simulink model "ekf2"  (R2023b)
settings: Solver=VariableStepAuto  StartTime=0.0  StopTime=Tend_slk  RelTol=1e-3
values from neighbouring files (symbols this model uses):
  IMU_w_b_bias = IMU_var_bias_matrix(:,2)    [ekf1_script.m]    (also in ekf2_script.m; ekf3_script.m)
  meas_pole = 15    [ekf1_script.m]    (also in ekf2_script.m; ekf3_script.m)
  P0_phth = diag([P0_ph,P0_th,P0_bias_wp,P0_bias_wq,P0_bias_wr])    [ekf2_script.m]    (also in ekf3_script.m)
  P0_ps = 100    [complementary_filter_script.m]    (also in ekf1_script.m; ekf2_script.m; ekf3_script.m)
  Q_phth = diag([q_ph,q_th,q_bias_w_b,q_bias_w_b,q_bias_w_b])    [ekf2_script.m]    (also in ekf3_script.m)
  q_ps = 100e-0    (= 100)    [complementary_filter_script.m]    (also in ekf1_script.m = 200; ekf2_script.m = 170; ekf3_script.m = 170)
  R_phth = diag([r_ph,r_th])    [ekf2_script.m]    (also in ekf3_script.m)
  r_ps = 600e+0    (= 600)    [complementary_filter_script.m]    (also in ekf1_script.m = 170; ekf2_script.m = 200; ekf3_script.m = 200)
  Ts_EKF_integr = 0.001    [complementary_filter_script.m]    (also in ekf1_script.m = 0.0001; ekf2_script.m = 0.0001; ekf3_script.m = 0.0001)
  Ts_EKF_meas = 0.01    [complementary_filter_script.m]    (also in ekf1_script.m; ekf2_script.m; ekf3_script.m)
  Ts_slk = 0.01    [complementary_filter_script.m]    (also in ekf1_script.m; ekf2_script.m; ekf3_script.m)
  x0_phth = [ph0;th0;bias_wp0;bias_wq0;bias_wr0]    [ekf2_script.m]    (also in ekf3_script.m)
  x0_ps = 0    [complementary_filter_script.m]    (also in ekf2_script.m; ekf3_script.m)
settings Model: Creator=teoma  LastModifiedBy=teoma

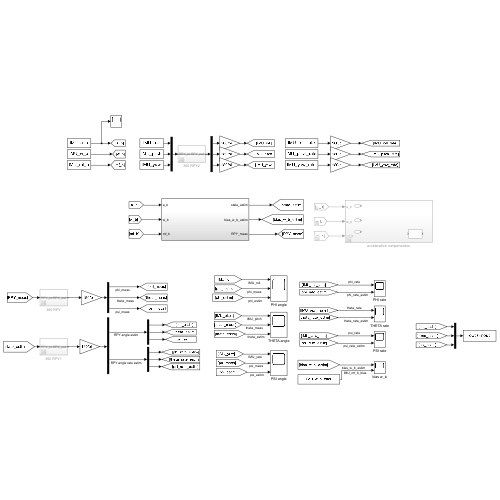
[thumbnail: Simulink's stored preview of the top-level diagram]
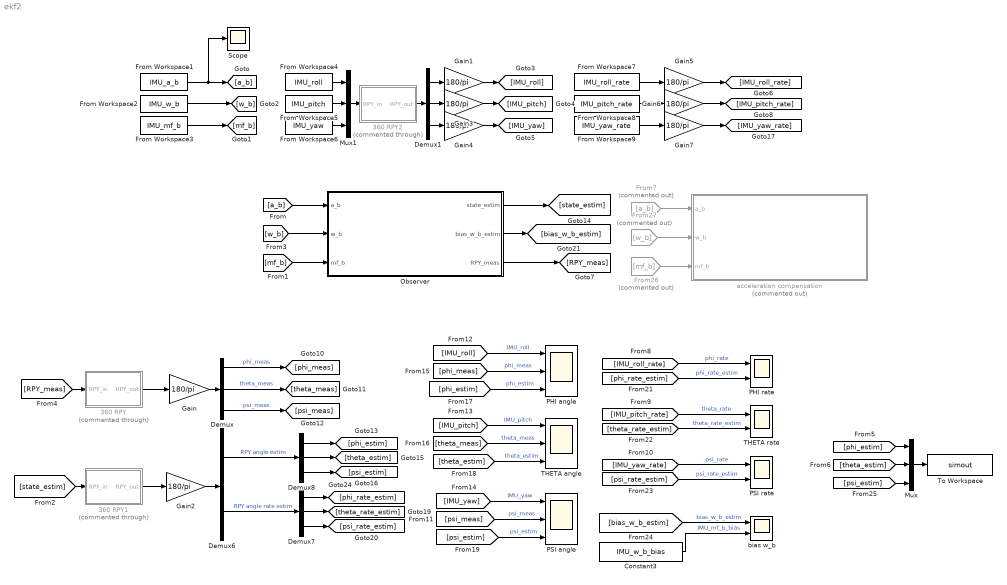
== system ekf2 ==
  360 RPY : Subsystem  Commented=through
  360 RPY1 : Subsystem  Commented=through
  360 RPY2 : Subsystem  Commented=through
  Constant3 : Constant  Value=IMU_w_b_bias
  Demux{,1,7..8} (4 alike) : Demux  Outputs=3
  Demux6 : Demux  Outputs=2
  From Workspace1 : FromWorkspace  VariableName=IMU_a_b  OutDataTypeStr=double  SampleTime=Ts_slk  Interpolate=off  OutputAfterFinalValue=Setting to zero
  From Workspace2 : FromWorkspace  VariableName=IMU_w_b  OutDataTypeStr=double  SampleTime=Ts_slk  Interpolate=off  OutputAfterFinalValue=Setting to zero
  From Workspace3 : FromWorkspace  VariableName=IMU_mf_b  OutDataTypeStr=double  SampleTime=Ts_slk  Interpolate=off  OutputAfterFinalValue=Setting to zero
  From Workspace4 : FromWorkspace  VariableName=IMU_roll  OutDataTypeStr=double  SampleTime=Ts_slk  Interpolate=off  OutputAfterFinalValue=Setting to zero
  From Workspace5 : FromWorkspace  VariableName=IMU_pitch  OutDataTypeStr=double  SampleTime=Ts_slk  Interpolate=off  OutputAfterFinalValue=Setting to zero
  From Workspace6 : FromWorkspace  VariableName=IMU_yaw  OutDataTypeStr=double  SampleTime=Ts_slk  Interpolate=off  OutputAfterFinalValue=Setting to zero
  From Workspace7 : FromWorkspace  VariableName=IMU_roll_rate  OutDataTypeStr=double  SampleTime=Ts_slk  Interpolate=off  OutputAfterFinalValue=Setting to zero
  From Workspace8 : FromWorkspace  VariableName=IMU_pitch_rate  OutDataTypeStr=double  SampleTime=Ts_slk  Interpolate=off  OutputAfterFinalValue=Setting to zero
  From Workspace9 : FromWorkspace  VariableName=IMU_yaw_rate  OutDataTypeStr=double  SampleTime=Ts_slk  Interpolate=off  OutputAfterFinalValue=Setting to zero
  From26 : From  Commented=on  GotoTag=mf_b
  From27 : From  Commented=on  GotoTag=w_b
  From7 : From  Commented=on  GotoTag=a_b
  Gain{,1..7} (8 alike) : Gain  Gain=180/pi
  Mux : Mux  Inputs=3
  Mux1 : Mux  Inputs=3
  Observer : Subsystem
  PHI angle : Scope  NumInputPorts=3
  PHI rate : Scope  NumInputPorts=2
  PSI angle : Scope  NumInputPorts=3
  PSI rate : Scope  NumInputPorts=2
  Scope : Scope
  THETA angle : Scope  NumInputPorts=3
  THETA rate : Scope  NumInputPorts=2
  To Workspace : ToWorkspace  VariableName=simout  SampleTime=-1
  acceleration compensation : Subsystem  Commented=on
  bias w_b : Scope  NumInputPorts=2
  wires:
  [a_b] -> Observer/1(a_b)
  Gain6/1 -> [IMU_pitch_rate]
  Observer/2(bias_w_b_estim) -> [bias_w_b_estim]
  [mf_b] -> Observer/3(mf_b)
  [IMU_roll] -> PHI angle/1  "IMU_roll"
  From Workspace9/1 -> Gain7/1
  Observer/3(RPY_meas) -> [RPY_meas]
  [IMU_yaw_rate] -> PSI rate/1  "psi_rate"
  [psi_estim] -> PSI angle/3  "psi_estim"
  Observer/1(state_estim) -> [state_estim]
  [w_b] -> Observer/2(w_b)
  From Workspace2/1 -> [w_b]
  [theta_estim] -> THETA angle/3  "theta_estim"
  [IMU_roll_rate] -> PHI rate/1  "phi_rate"
  [phi_meas] -> PHI angle/2  "phi_meas"
  Constant3/1 -> bias w_b/2  "IMU_mf_b_bias"
  From Workspace1/1 -> [a_b], Scope/1
  From Workspace7/1 -> Gain5/1
  [IMU_yaw] -> PSI angle/1  "IMU_yaw"
  [phi_estim] -> PHI angle/3  "phi_estim"
  [theta_rate_estim] -> THETA rate/2  "theta_rate_estim"
  [psi_rate_estim] -> PSI rate/2  "psi_rate_estim"
  [IMU_pitch_rate] -> THETA rate/1  "theta_rate"
  Gain7/1 -> [IMU_yaw_rate]
  [theta_meas] -> THETA angle/2  "theta_meas"
  [IMU_pitch] -> THETA angle/1  "IMU_pitch"
  [psi_meas] -> PSI angle/2  "psi_meas"
  Gain5/1 -> [IMU_roll_rate]
  From Workspace8/1 -> Gain6/1
  [phi_rate_estim] -> PHI rate/2  "phi_rate_estim"
  From Workspace3/1 -> [mf_b]
  [bias_w_b_estim] -> bias w_b/1  "bias_w_b_estim"
  Mux/1 -> To Workspace/1
  [phi_estim] -> Mux/1
  [theta_estim] -> Mux/2
  [psi_estim] -> Mux/3
  From27/1 -> acceleration compensation/2(w_b)
  From26/1 -> acceleration compensation/3(mf_b)
  From7/1 -> acceleration compensation/1(a_b)
  360 RPY1/1(RPY_out) -> Gain2/1
  Demux6/1 -> Demux8/1  "RPY angle estim"
  Demux6/2 -> Demux7/1  "RPY angle rate estim"
  Demux/2 -> [theta_meas]  "theta_meas"
  Gain/1 -> Demux/1
  Demux7/2 -> [theta_rate_estim]
  Demux8/3 -> [psi_estim]
  Demux8/2 -> [theta_estim]
  Demux7/3 -> [psi_rate_estim]
  Demux/1 -> [phi_meas]  "phi_meas"
  Gain2/1 -> Demux6/1
  Demux8/1 -> [phi_estim]
  Demux7/1 -> [phi_rate_estim]
  360 RPY/1(RPY_out) -> Gain/1
  Demux/3 -> [psi_meas]  "psi_meas"
  [state_estim] -> 360 RPY1/1(RPY_in)
  [RPY_meas] -> 360 RPY/1(RPY_in)
  Mux1/1 -> 360 RPY2/1(RPY_in)
  Demux1/1 -> Gain1/1
  From Workspace4/1 -> Mux1/1
  Gain1/1 -> [IMU_roll]
  Gain3/1 -> [IMU_pitch]
  Demux1/2 -> Gain3/1
  Demux1/3 -> Gain4/1
  From Workspace5/1 -> Mux1/2
  Gain4/1 -> [IMU_yaw]
  From Workspace6/1 -> Mux1/3
  360 RPY2/1(RPY_out) -> Demux1/1

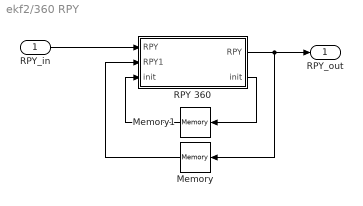
== system ekf2/360 RPY ==
  RPY_in : Inport
  Memory : Memory
  Memory1 : Memory
  RPY 360 : MATLAB Function  TreatAsAtomicUnit=on
  RPY_out : Outport
  wires:
  Memory/1 -> RPY 360/2(RPY1)
  Memory1/1 -> RPY 360/3("init ")
  RPY 360/2(init) -> Memory1/1
  RPY 360/1(RPY) -> Memory/1, RPY_out/1
  RPY_in/1 -> RPY 360/1("RPY ")

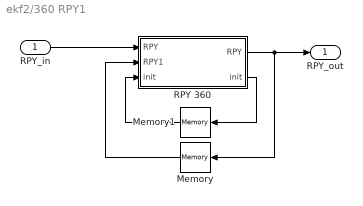
== system ekf2/360 RPY1 ==
  RPY_in : Inport
  Memory : Memory
  Memory1 : Memory
  RPY 360 : MATLAB Function  TreatAsAtomicUnit=on
  RPY_out : Outport
  wires:
  Memory/1 -> RPY 360/2(RPY1)
  Memory1/1 -> RPY 360/3("init ")
  RPY 360/2(init) -> Memory1/1
  RPY 360/1(RPY) -> Memory/1, RPY_out/1
  RPY_in/1 -> RPY 360/1("RPY ")

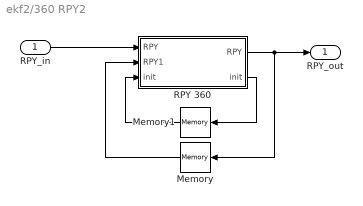
== system ekf2/360 RPY2 ==
  RPY_in : Inport
  Memory : Memory
  Memory1 : Memory
  RPY 360 : MATLAB Function  TreatAsAtomicUnit=on
  RPY_out : Outport
  wires:
  Memory/1 -> RPY 360/2(RPY1)
  Memory1/1 -> RPY 360/3("init ")
  RPY 360/2(init) -> Memory1/1
  RPY 360/1(RPY) -> Memory/1, RPY_out/1
  RPY_in/1 -> RPY 360/1("RPY ")

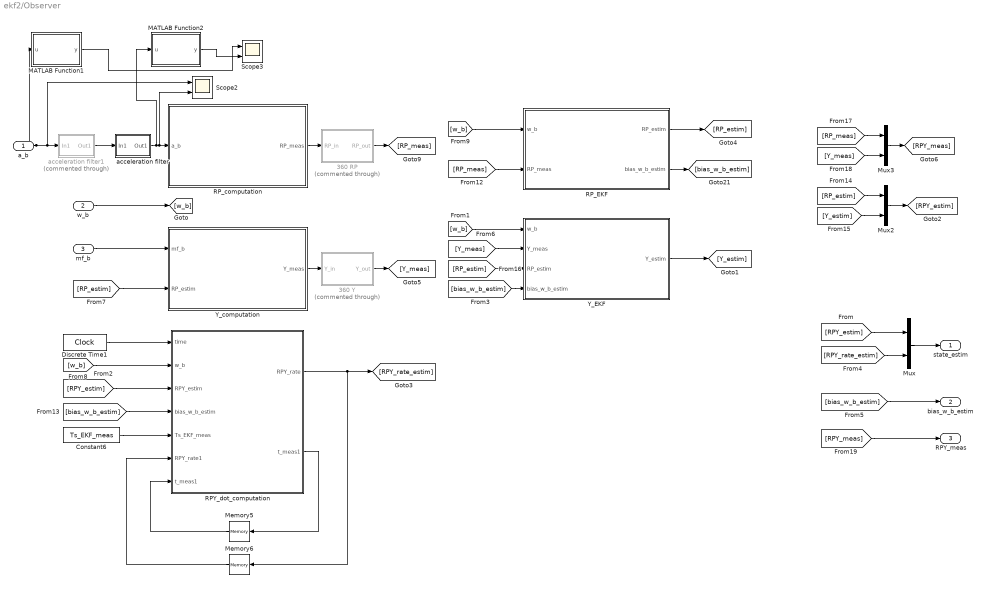
== system ekf2/Observer ==
  a_b : Inport
  w_b : Inport  Port=2
  mf_b : Inport  Port=3
  360 RP : Subsystem  Commented=through
  360 Y : Subsystem  Commented=through
  Constant6 : Constant  Value=Ts_EKF_meas
  Discrete Time1 : DigitalClock  SampleTime=Ts_slk
  MATLAB Function1 : MATLAB Function  TreatAsAtomicUnit=on
  MATLAB Function2 : MATLAB Function  TreatAsAtomicUnit=on
  Memory5 : Memory
  Memory6 : Memory
  Mux : Mux  Inputs=2
  Mux2 : Mux  Inputs=2
  Mux3 : Mux  Inputs=2
  RPY_dot_computation : MATLAB Function  TreatAsAtomicUnit=on
  RP_EKF : Subsystem
  RP_computation : MATLAB Function  TreatAsAtomicUnit=on
  Scope2 : Scope  NumInputPorts=2
  Scope3 : Scope  NumInputPorts=2
  Y_EKF : Subsystem
  Y_computation : MATLAB Function  TreatAsAtomicUnit=on
  acceleration filter : Subsystem  mask{p=meas_pole}
      mask prompts: p "pole (p)"
  acceleration filter1 : Subsystem  Commented=through  mask{p=5}
      mask prompts: p "pole (p)"
  state_estim : Outport
  bias_w_b_estim : Outport  Port=2
  RPY_meas : Outport  Port=3
  wires:
  Memory5/1 -> RPY_dot_computation/7("t_meas1 ")
  Discrete Time1/1 -> RPY_dot_computation/1(time)
  RPY_dot_computation/2(t_meas1) -> Memory5/1
  [w_b] -> RPY_dot_computation/2(w_b)
  Memory6/1 -> RPY_dot_computation/6(RPY_rate1)
  RPY_dot_computation/1(RPY_rate) -> Memory6/1, [RPY_rate_estim]
  Constant6/1 -> RPY_dot_computation/5(Ts_EKF_meas)
  [RPY_estim] -> RPY_dot_computation/3(RPY_estim)
  [bias_w_b_estim] -> RPY_dot_computation/4(bias_w_b_estim)
  [RPY_estim] -> Mux/1
  [RPY_rate_estim] -> Mux/2
  Mux/1 -> state_estim/1
  [bias_w_b_estim] -> bias_w_b_estim/1
  [RPY_meas] -> RPY_meas/1
  RP_EKF/2(bias_w_b_estim) -> [bias_w_b_estim]
  [RP_estim] -> Y_computation/2(RP_estim)
  [Y_meas] -> Y_EKF/2(Y_meas)
  Y_computation/1(Y_meas) -> 360 Y/1(Y_in)
  RP_EKF/1(RP_estim) -> [RP_estim]
  [w_b] -> Y_EKF/1(w_b)
  RP_computation/1(RP_meas) -> 360 RP/1(RP_in)
  [RP_meas] -> RP_EKF/2(RP_meas)
  [w_b] -> RP_EKF/1(w_b)
  Y_EKF/1(Y_estim) -> [Y_estim]
  mf_b/1 -> Y_computation/1(mf_b)
  w_b/1 -> [w_b]
  [bias_w_b_estim] -> Y_EKF/4(bias_w_b_estim)
  [RP_estim] -> Mux2/1
  [Y_estim] -> Mux2/2
  Mux2/1 -> [RPY_estim]
  [RP_estim] -> Y_EKF/3(RP_estim)
  [RP_meas] -> Mux3/1
  Mux3/1 -> [RPY_meas]
  [Y_meas] -> Mux3/2
  MATLAB Function1/1(y) -> Scope3/1
  a_b/1 -> Scope2/1, acceleration filter1/1(In1), MATLAB Function1/1(u)
  MATLAB Function2/1(y) -> Scope3/2
  acceleration filter/1(Out1) -> MATLAB Function2/1(u), Scope2/2, RP_computation/1(a_b)
  360 Y/1(Y_out) -> [Y_meas]
  360 RP/1(RP_out) -> [RP_meas]
  acceleration filter1/1(Out1) -> acceleration filter/1(In1)

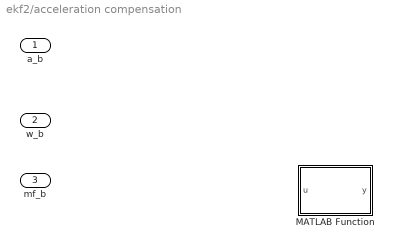
== system ekf2/acceleration compensation ==
  a_b : Inport
  w_b : Inport  Port=2
  mf_b : Inport  Port=3
  MATLAB Function : MATLAB Function  TreatAsAtomicUnit=on

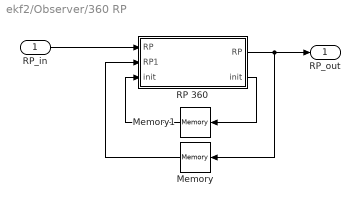
== system ekf2/Observer/360 RP ==
  RP_in : Inport
  Memory : Memory
  Memory1 : Memory
  RP 360 : MATLAB Function  TreatAsAtomicUnit=on
  RP_out : Outport
  wires:
  RP_in/1 -> RP 360/1("RP ")
  RP 360/1(RP) -> Memory/1, RP_out/1
  Memory/1 -> RP 360/2(RP1)
  RP 360/2(init) -> Memory1/1
  Memory1/1 -> RP 360/3("init ")

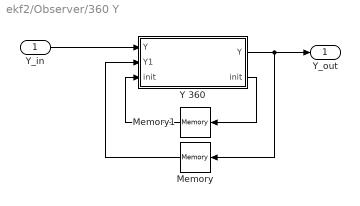
== system ekf2/Observer/360 Y ==
  Y_in : Inport
  Memory : Memory
  Memory1 : Memory
  Y 360 : MATLAB Function  TreatAsAtomicUnit=on
  Y_out : Outport
  wires:
  Y_in/1 -> Y 360/1("Y ")
  Y 360/1(Y) -> Memory/1, Y_out/1
  Memory/1 -> Y 360/2(Y1)
  Y 360/2(init) -> Memory1/1
  Memory1/1 -> Y 360/3("init ")

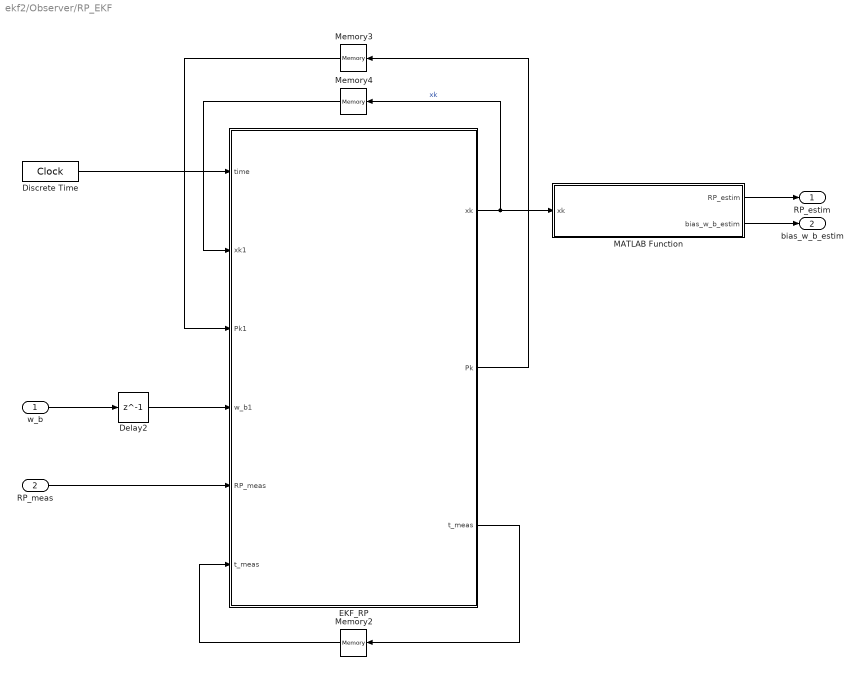
== system ekf2/Observer/RP_EKF ==
  w_b : Inport
  RP_meas : Inport  Port=2
  Delay2 : Delay  DelayLength=1  SampleTime=Ts_EKF_meas
  Discrete Time : DigitalClock  SampleTime=Ts_slk
  EKF_RP : MATLAB Function  TreatAsAtomicUnit=on
  MATLAB Function : MATLAB Function  TreatAsAtomicUnit=on
  Memory2 : Memory
  Memory3 : Memory  InitialCondition=P0_phth
  Memory4 : Memory  InitialCondition=x0_phth
  RP_estim : Outport
  bias_w_b_estim : Outport  Port=2
  wires:
  w_b/1 -> Delay2/1
  EKF_RP/2(Pk) -> Memory3/1
  Memory2/1 -> EKF_RP/6("t_meas ")
  EKF_RP/3(t_meas) -> Memory2/1
  RP_meas/1 -> EKF_RP/5(RP_meas)
  Discrete Time/1 -> EKF_RP/1(time)
  Memory3/1 -> EKF_RP/3(Pk1)
  Delay2/1 -> EKF_RP/4(w_b1)
  Memory4/1 -> EKF_RP/2(xk1)
  EKF_RP/1(xk) -> Memory4/1, MATLAB Function/1(xk)  "xk"
  MATLAB Function/1(RP_estim) -> RP_estim/1
  MATLAB Function/2(bias_w_b_estim) -> bias_w_b_estim/1

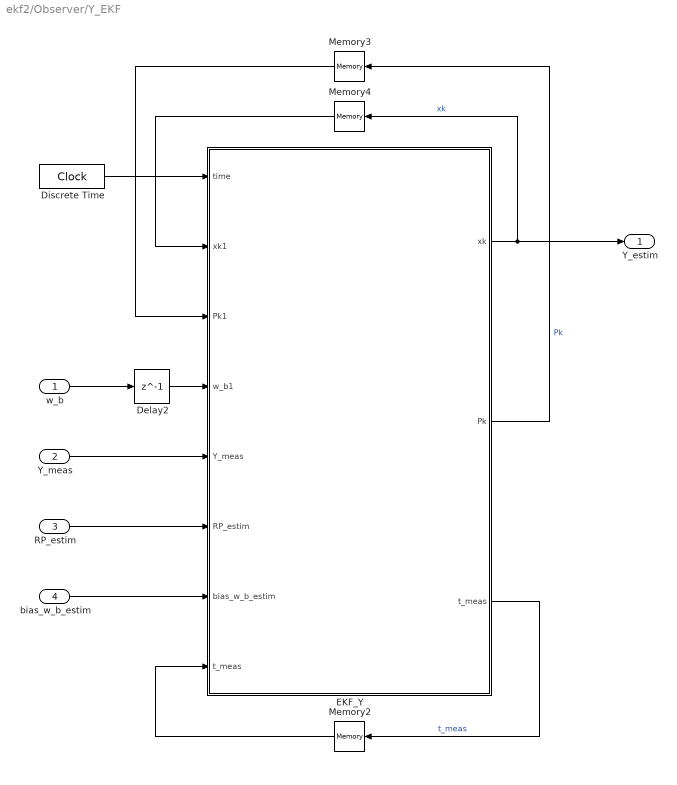
== system ekf2/Observer/Y_EKF ==
  w_b : Inport
  Y_meas : Inport  Port=2
  RP_estim : Inport  Port=3
  bias_w_b_estim : Inport  Port=4
  Delay2 : Delay  DelayLength=1  SampleTime=Ts_EKF_meas
  Discrete Time : DigitalClock  SampleTime=Ts_slk
  EKF_Y : MATLAB Function  TreatAsAtomicUnit=on
  Memory2 : Memory
  Memory3 : Memory  InitialCondition=ones(1,1)*P0_ps
  Memory4 : Memory  InitialCondition=ones(1,1)*x0_ps
  Y_estim : Outport
  wires:
  w_b/1 -> Delay2/1
  EKF_Y/2(Pk) -> Memory3/1  "Pk"
  Memory2/1 -> EKF_Y/8("t_meas ")
  EKF_Y/3(t_meas) -> Memory2/1  "t_meas"
  Y_meas/1 -> EKF_Y/5(Y_meas)
  Discrete Time/1 -> EKF_Y/1(time)
  Memory3/1 -> EKF_Y/3(Pk1)
  Delay2/1 -> EKF_Y/4(w_b1)
  Memory4/1 -> EKF_Y/2(xk1)
  EKF_Y/1(xk) -> Memory4/1, Y_estim/1  "xk"
  bias_w_b_estim/1 -> EKF_Y/7(bias_w_b_estim)
  RP_estim/1 -> EKF_Y/6(RP_estim)

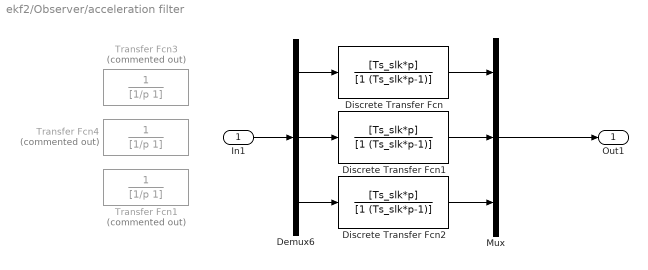
== system ekf2/Observer/acceleration filter ==
  In1 : Inport
  Demux6 : Demux  Outputs=3
  Discrete Transfer Fcn : DiscreteTransferFcn  Numerator=[Ts_slk*p]  Denominator=[1 (Ts_slk*p-1)]
  Discrete Transfer Fcn1 : DiscreteTransferFcn  Numerator=[Ts_slk*p]  Denominator=[1 (Ts_slk*p-1)]
  Discrete Transfer Fcn2 : DiscreteTransferFcn  Numerator=[Ts_slk*p]  Denominator=[1 (Ts_slk*p-1)]
  Mux : Mux  Inputs=3
  Transfer Fcn1 : TransferFcn  Commented=on  Denominator=[1/p 1]
  Transfer Fcn3 : TransferFcn  Commented=on  Denominator=[1/p 1]
  Transfer Fcn4 : TransferFcn  Commented=on  Denominator=[1/p 1]
  Out1 : Outport
  wires:
  Discrete Transfer Fcn1/1 -> Mux/2
  Demux6/3 -> Discrete Transfer Fcn2/1
  Mux/1 -> Out1/1
  Discrete Transfer Fcn2/1 -> Mux/3
  Discrete Transfer Fcn/1 -> Mux/1
  In1/1 -> Demux6/1
  Demux6/1 -> Discrete Transfer Fcn/1
  Demux6/2 -> Discrete Transfer Fcn1/1

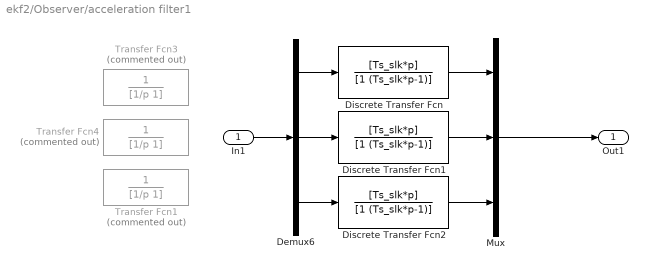
== system ekf2/Observer/acceleration filter1 ==
  In1 : Inport
  Demux6 : Demux  Outputs=3
  Discrete Transfer Fcn : DiscreteTransferFcn  Numerator=[Ts_slk*p]  Denominator=[1 (Ts_slk*p-1)]
  Discrete Transfer Fcn1 : DiscreteTransferFcn  Numerator=[Ts_slk*p]  Denominator=[1 (Ts_slk*p-1)]
  Discrete Transfer Fcn2 : DiscreteTransferFcn  Numerator=[Ts_slk*p]  Denominator=[1 (Ts_slk*p-1)]
  Mux : Mux  Inputs=3
  Transfer Fcn1 : TransferFcn  Commented=on  Denominator=[1/p 1]
  Transfer Fcn3 : TransferFcn  Commented=on  Denominator=[1/p 1]
  Transfer Fcn4 : TransferFcn  Commented=on  Denominator=[1/p 1]
  Out1 : Outport
  wires:
  Discrete Transfer Fcn1/1 -> Mux/2
  Demux6/3 -> Discrete Transfer Fcn2/1
  Mux/1 -> Out1/1
  Discrete Transfer Fcn2/1 -> Mux/3
  Discrete Transfer Fcn/1 -> Mux/1
  In1/1 -> Demux6/1
  Demux6/1 -> Discrete Transfer Fcn/1
  Demux6/2 -> Discrete Transfer Fcn1/1

== matlab function ekf2/Observer/RP_EKF/MATLAB Function ==
  data: xk input; RP_estim output; bias_w_b_estim output
function [RP_estim, bias_w_b_estim] = state_extraction(xk)

RP_estim        = xk(1:2,1);
bias_w_b_estim  = xk(3:5,1);
end

== matlab function ekf2/acceleration compensation/MATLAB Function ==
  data: u input; y output
function y = GCF(u)

y = u;

== matlab function ekf2/360 RPY2/RPY 360 ==
  data: RPY input; RPY output; RPY1 input; init output; init input
function [RPY,init] = RPY_360(RPY,RPY1,init)
if init < 2 
    if init == 0
        init = 1;
        RPY1 = RPY;
    elseif init == 1
        if (RPY - RPY1)'*(RPY - RPY1) > 0.01
            init = 2;
            RPY1 = RPY;
        end
    end
end

% - pi <= PHI <= + pi PHI uses atan2()
if abs(RPY(1) - RPY1(1)) > pi*0.99
    RPY(1) = RPY(1) + sign(RPY1(1))*(2*pi);
end
% - pi/2 <= THETA <= + pi/2 THETA uses asin()
if abs(RPY(2) - RPY1(2)) > pi/2*0.99
    RPY(2) = RPY(2) + sign(RPY1(2))*(2*pi);
end
% - pi <= PSI <= + pi PSI uses atan2()
if abs(RPY(3) - RPY1(3)) > pi*0.99
    RPY(3) = RPY(3) + sign(RPY1(3))*(2*pi);
end
end

== matlab function ekf2/Observer/RPY_dot_computation ==
  data: time input; w_b input; RPY_estim input; bias_w_b_estim input; Ts_EKF_meas input; RPY_rate1 input; RPY_rate output; t_meas1 input; t_meas1 output
function [RPY_rate,t_meas1] = RPY_dot_computation(time,w_b,RPY_estim,bias_w_b_estim,Ts_EKF_meas,RPY_rate1,t_meas1)

if time - t_meas1 >= Ts_EKF_meas || time == 0
    wp          =       w_b(1,1);               % p-dir of angular velocity w
    wq          =       w_b(2,1);               % q-dir of angular velocity w
    wr          =       w_b(3,1);               % r-dir of angular velocity w

    phi         =       RPY_estim(1,1);         % roll angle (rad)
    theta       =       RPY_estim(2,1);         % pitch angle (rad)
    psi         =       RPY_estim(3,1);         % yaw angle (rad)  
    bias_wp     =       bias_w_b_estim(1,1)*0;    % bias of p-dir of angular velocity w
    bias_wq     =       bias_w_b_estim(2,1)*0;    % bias of q-dir of angular velocity w
    bias_wr     =       bias_w_b_estim(3,1)*0;   % bias of r-dir of angular velocity w

    cph         =       cos(phi);
    cth         =       cos(theta);
    cps         =       cos(psi);
    sph         =       sin(phi);
    sth         =       sin(theta);
    sps         =       sin(psi);
    tth         =       sth/cth;

    % integration step
    t_meas1 = time;
    W_eta = [1,    sph*tth,    cph*tth;
             0,    cph,        -sph;
             0,    sph/cth,    cph/cth;];
    w_b_corrected = [wp-bias_wp; wq-bias_wq; wr-bias_wr;];
    RPY_rate = W_eta*w_b_corrected;
else
    RPY_rate = RPY_rate1;
end
end

== matlab function ekf2/360 RPY/RPY 360 ==
  data: RPY input; RPY output; RPY1 input; init output; init input
function [RPY,init] = RPY_360(RPY,RPY1,init)
if init < 2 
    if init == 0
        init = 1;
        RPY1 = RPY;
    elseif init == 1
        if (RPY - RPY1)'*(RPY - RPY1) > 0.01
            init = 2;
            RPY1 = RPY;
        end
    end
end

% - pi <= PHI <= + pi PHI uses atan2()
if abs(RPY(1) - RPY1(1)) > pi*0.99
    RPY(1) = RPY(1) + sign(RPY1(1))*(2*pi);
end
% - pi/2 <= THETA <= + pi/2 THETA uses asin()
if abs(RPY(2) - RPY1(2)) > pi/2*0.99
    RPY(2) = RPY(2) + sign(RPY1(2))*(2*pi);
end
% - pi <= PSI <= + pi PSI uses atan2()
if abs(RPY(3) - RPY1(3)) > pi*0.99
    RPY(3) = RPY(3) + sign(RPY1(3))*(2*pi);
end
end

== matlab function ekf2/Observer/360 Y/Y 360 ==
  data: Y input; Y output; Y1 input; init output; init input
function [Y,init] = Y_360(Y,Y1, init)
if init < 2 
    if init == 0
        init = 1;
        Y1 = Y;
    elseif init == 1
        if (Y - Y1)'*(Y - Y1) > 0.01
            init = 2;
            Y1 = Y;
        end
    end
end

% - pi <= PSI <= + pi PSI uses atan2()
if abs(Y - Y1) > pi*0.99
    Y = Y + sign(Y1)*(2*pi);
end

== matlab function ekf2/Observer/360 RP/RP 360 ==
  data: RP input; RP output; RP1 input; init output; init input
function [RP,init] = RP_360(RP,RP1, init)
if init < 2 
    if init == 0
        init = 1;
        RP1 = RP;
    elseif init == 1
        if (RP - RP1)'*(RP - RP1) > 0.01
            init = 2;
            RP1 = RP;
        end
    end
end

% - pi <= PHI <= + pi PHI uses atan2()
if abs(RP(1) - RP1(1)) > pi*0.99
    RP(1) = RP(1) + sign(RP1(1))*(2*pi);
end
% - pi/2 <= THETA <= + pi/2 THETA uses asin()
if abs(RP(2) - RP1(2)) > pi/2*0.99
    RP(2) = RP(2) + sign(RP1(2))*(2*pi);
end

end

== matlab function ekf2/Observer/Y_computation ==
  data: mf_b input; RP_estim input; Y_meas output
function Y_meas    = Y_computation(mf_b,RP_estim)
% description:
% - a_b             = measured linear acceleration in body-frame
% - w_b             = measured angular velocity in body-frame
% - mf_b            = measured magnetic field in body-frame
% - mf              = measured magnetic field in body-inertia
% - a_b_disturbe    = linear velocity measurement-noise
% - w_b_disturbe    = angular velocity measurement-noise
% - mf_b_disturbe   = magnetic field measurement-noise

% -------------------------------------------------------------------------------------------
% observation: the following computation works only if the angles
% phi,theta,psy are withing angles (-pi/2,+pi/2) (this is an open set, pi/2 is excluded)
% -------------------------------------------------------------------------------------------

ph_estim = RP_estim(1,1);
th_estim = RP_estim(2,1);

sph = sin(ph_estim);
cph = cos(ph_estim);

sth = sin(th_estim);
cth = cos(th_estim);

ps_meas_num   = mf_b(3)*sph - mf_b(2)*cph;
ps_meas_den = mf_b(1)*cth + mf_b(2)*sth*sph + mf_b(3)*sth*cph;
ps_meas = atan2(ps_meas_num, ps_meas_den);

Y_meas = ps_meas;
end

== matlab function ekf2/360 RPY1/RPY 360 ==
  data: RPY input; RPY output; RPY1 input; init output; init input
function [RPY,init] = RPY_360(RPY,RPY1,init)
if init < 2 
    if init == 0
        init = 1;
        RPY1 = RPY;
    elseif init == 1
        if (RPY - RPY1)'*(RPY - RPY1) > 0.01
            init = 2;
            RPY1 = RPY;
        end
    end
end

% - pi <= PHI <= + pi PHI uses atan2()
if abs(RPY(1) - RPY1(1)) > pi*0.99
    RPY(1) = RPY(1) + sign(RPY1(1))*(2*pi);
end
% - pi/2 <= THETA <= + pi/2 THETA uses asin()
if abs(RPY(2) - RPY1(2)) > pi/2*0.99
    RPY(2) = RPY(2) + sign(RPY1(2))*(2*pi);
end
% - pi <= PSI <= + pi PSI uses atan2()
if abs(RPY(3) - RPY1(3)) > pi*0.99
    RPY(3) = RPY(3) + sign(RPY1(3))*(2*pi);
end
end

== matlab function ekf2/Observer/Y_EKF/EKF_Y ==
  data: time input; xk1 input size=[1,1]; Pk1 input size=[1,1]; w_b1 input; Y_meas input; RP_estim input; bias_w_b_estim input; t_meas input; q_ps parameter; xk output size=[1,1]; Pk output; t_meas output; r_ps parameter; Ts_EKF_integr parameter; Ts_EKF_meas parameter
function [xk,Pk,t_meas] = EKF_Y(time,xk1,Pk1,w_b1,Y_meas,RP_estim,bias_w_b_estim,t_meas,q_ps,r_ps,Ts_EKF_integr,Ts_EKF_meas)

if time - t_meas >= Ts_EKF_meas
    t_meas = time;
    Q = q_ps;
    R = r_ps;

  % INTEGRATION STEP
    % initial condition
    xt1         =       xk1;                        % initial condition for the state
    Pt1         =       Pk1;                        % initial condition for matrix P

    wp1         =       w_b1(1,1);                  % past value of the p-dir of angular velocity w
    wq1         =       w_b1(2,1);                  % past value of the q-dir of angular velocity w
    wr1         =       w_b1(3,1);                  % past value of the r-dir of angular velocity w

    phi         =       RP_estim(1,1);              % estimate of roll angle (rad)
    theta       =       RP_estim(2,1);              % estimate of pitch angle (rad)  

    bias_wp     =       bias_w_b_estim(1,1);        % estimate of bias of p-dir of angular velocity w
    bias_wq     =       bias_w_b_estim(2,1);        % estimate of bias of q-dir of angular velocity w
    bias_wr     =       bias_w_b_estim(3,1);        % estimate of bias of r-dir of angular velocity w
    % integration loop
    Nstep       = floor(Ts_EKF_meas/Ts_EKF_integr); % number of integration steps to performe in the t_meas time windows
    xt          = zeros(1,1);
    Pt          = zeros(1,1);
    for i = 1:1:Nstep
        % state extraction
            psi         =       xt1(1,1);           % roll angle (rad)
        
            cph         =       cos(phi);
            cth         =       cos(theta);
            cps         =       cos(psi);
            sph         =       sin(phi);
            sth         =       sin(theta);
            sps         =       sin(psi);
            tth         =       sth/cth;
        % integration
            Mf = [0,    sph/cth,    cph/cth,    0,  0,  0;];
            Z1 = [wp1-bias_wp; wq1-bias_wq; wr1-bias_wr; bias_wp; bias_wq; bias_wr;];
            f = Mf*Z1;
            xt = xt1 + Ts_EKF_integr*f;
        
            At1 = 0;
            Pt = Pt1 + Ts_EKF_integr*(At1*Pt1 + Pt1*At1' + Q);
        % house keeping
            xt1 = xt;
            Pt1 = Pt;
    end
  % MEASUREMENT STEP
    Ck = [eye(1)];
    Lk = Pt*Ck'/(Ck*Pt*Ck' + R);
    xk = xt + Lk*(Y_meas - Ck*xt);
    Pk = (eye(1) - Lk*Ck)*Pt;
else
    xk = xk1;
    Pk = Pk1;
end
end

== matlab function ekf2/Observer/RP_computation ==
  data: a_b input; RP_meas output
function RP_meas    = RP_computation(a_b)
% description:
% - a_b             = measured linear acceleration in body-frame
% - w_b             = measured angular velocity in body-frame
% - mf_b            = measured magnetic field in body-frame
% - mf              = measured magnetic field in body-inertia
% - a_b_disturbe    = linear velocity measurement-noise
% - w_b_disturbe    = angular velocity measurement-noise
% - mf_b_disturbe   = magnetic field measurement-noise

% -------------------------------------------------------------------------------------------
% observation: the following computation works only if the angles
% phi,theta,psy are withing angles (-pi/2,+pi/2) (this is an open set, pi/2 is excluded)
% -------------------------------------------------------------------------------------------

a_b = -1*a_b;       % need to adjust the sign to use atan2() function correctly

% phi computation
ph_meas = atan2(a_b(2), a_b(3));
sph = sin(ph_meas);
cph = cos(ph_meas);

% theta computation
th_meas = atan2(-a_b(1), (a_b(2)*sph + a_b(3)*cph));

RP_meas = [ph_meas;th_meas];

== matlab function ekf2/Observer/RP_EKF/EKF_RP ==
  data: time input; xk1 input; Pk1 input; w_b1 input; RP_meas input; t_meas input; Q_phth parameter; xk output; Pk output; t_meas output; R_phth parameter; Ts_EKF_integr parameter; Ts_EKF_meas parameter
function [xk,Pk,t_meas] = EKF_RP(time,xk1,Pk1,w_b1,RP_meas,t_meas,Q_phth,R_phth,Ts_EKF_integr,Ts_EKF_meas)

if time - t_meas >= Ts_EKF_meas
    t_meas = time;
    Q = Q_phth;
    R = R_phth;

  % INTEGRATION STEP
    % initial condition
    xt1         =       xk1;                        % initial condition for the state
    Pt1         =       Pk1;                        % initial condition for matrix P
    wp1         =       w_b1(1,1);                  % past value of the p-dir of angular velocity w
    wq1         =       w_b1(2,1);                  % past value of the q-dir of angular velocity w
    wr1         =       w_b1(3,1);                  % past value of the r-dir of angular velocity w
    % integration loop
    Nstep       = floor(Ts_EKF_meas/Ts_EKF_integr); % number of integration steps to performe in the t_meas time windows
    xt          = zeros(5,1);
    Pt          = zeros(5,5);
    for i = 1:1:Nstep
        % state extraction
            phi         =       xt1(1,1);           % roll angle (rad)
            theta       =       xt1(2,1);           % pitch angle (rad)  
            bias_wp     =       xt1(3,1);           % bias of p-dir of angular velocity w
            bias_wq     =       xt1(4,1);           % bias of q-dir of angular velocity w
            bias_wr     =       xt1(5,1);           % bias of r-dir of angular velocity w
        
            cph         =       cos(phi);
            cth         =       cos(theta);
            sph         =       sin(phi);
            sth         =       sin(theta);
            tth         =       sth/cth;
        % integration
            Mf = [1,    sph*tth,    cph*tth,    0,  0,  0;
                  0,    cph,        -sph,       0,  0,  0;
                  0,    0,          0,          0,  0,  0;
                  0,    0,          0,          0,  0,  0;
                  0,    0,          0,          0,  0,  0;];
            Z1 = [wp1-bias_wp; wq1-bias_wq; wr1-bias_wr; bias_wp; bias_wq; bias_wr;];
            f = Mf*Z1;
            xt = xt1 + Ts_EKF_integr*f;
        
            A1 = [cph*tth*(wq1-bias_wq)-sph*tth*(wr1-bias_wr),(sph*(wq1-bias_wq)+cph*(wr1-bias_wr))/cth^2,  -1, -sph*tth,   -cph*tth;];
            A2 = [-sph*(wq1-bias_wq)-cph*(wr1-bias_wr),  0,  0,  -cph,   sph;];
            A3 = [0,  0,  0,  0,  0;];
            A4 = [0,  0,  0,  0,  0;];
            A5 = [0,  0,  0,  0,  0;];
            At1 = [A1; A2; A3; A4; A5;];
            Pt = Pt1 + Ts_EKF_integr*(At1*Pt1 + Pt1*At1' + Q);
        % house keeping
            xt1 = xt;
            Pt1 = Pt;
    end
  % MEASUREMENT STEP
    Ck = [eye(2),zeros(2,3)];
    Lk = Pt*Ck'/(Ck*Pt*Ck' + R);
    xk = xt + Lk*(RP_meas - Ck*xt);
    Pk = (eye(5) - Lk*Ck)*Pt;
else
    xk = xk1;
    Pk = Pk1;
end
end

== matlab function ekf2/Observer/MATLAB Function1 ==
  data: u input; y output
function y = fcn(u)

y = sqrt(u(1)^2 + u(2)^2 + u(3)^2);

== matlab function ekf2/Observer/MATLAB Function2 ==
  data: u input; y output
function y = fcn(u)

y = sqrt(u(1)^2 + u(2)^2 + u(3)^2);
